simulink model "object_tracker_for_demo"  (Simulink 6.4)
settings: Solver=FixedStepDiscrete  StartTime=0.0  StopTime=inf  RelTol=1e-3
StartFcn:
  | ppo_start
StopFcn:
  | ppo_stop
model workspace: external: M-Code (data not in the file)
undefined symbols (not defined in the file or in its folder): Kanade, line_row, Lucas, Rec, SDTV
libraries: dspmtrx3 x11, viptextngfix x9, vipsnks x5, vipconversions x3, vipanalysis x3, vipgeotforms x3, simulink x2, dspwin32 x1, vipstatistics x1, vipmisc x1, dspindex x1, imaqlib x1
settings Model: Creator=don  LastModifiedBy=Raza  ExtModeAutoUpdateStatusClock=off
settings DataIOCC: LimitDataPoints=off  SaveOutput=off  SignalLogging=off  SaveTime=off  SignalLoggingName=sigsOut
settings OptimizationCC: BufferReusableBoundary=off
settings DebuggingCC: AlgebraicLoopMsg=none  CheckExecutionContextPreStartOutputMsg=on  CheckExecutionContextRuntimeOutputMsg=on  SolverPrmCheckMsg=none  SigSpecEnsureSampleTimeMsg=none  ParameterPrecisionLossMsg=none  BusObjectLabelMismatch=none  StrictBusMsg=None
settings HardwareCC: TargetHWDeviceType=32-bit Generic  ProdEqTarget=off

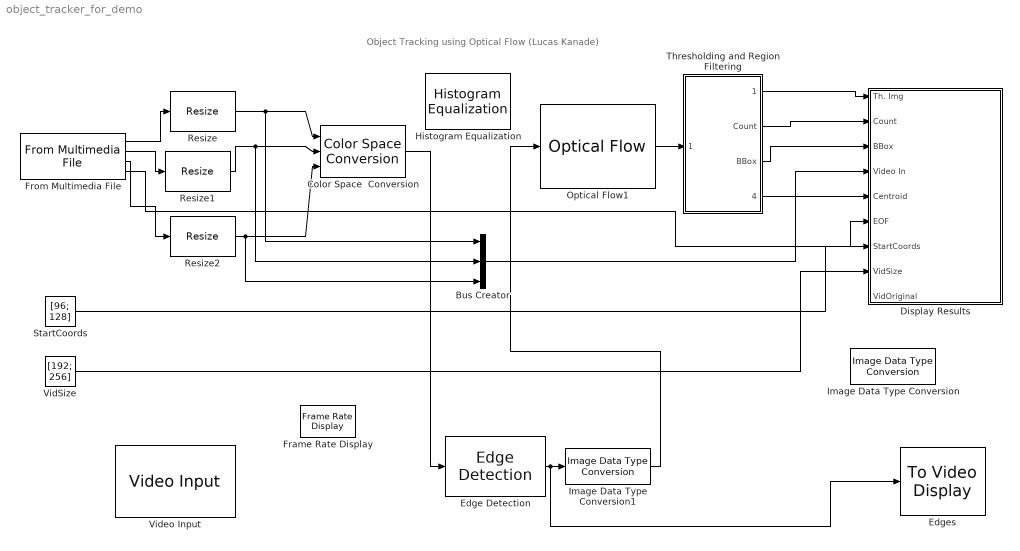
== system object_tracker_for_demo ==
  note: Object Tracking using Optical Flow (Lucas Kanade)
  Bus Creator : BusCreator  Inputs=3
  Color Space  Conversion : vipconversions/Color Space  Conversion  conversion=R'G'B' to intensity  wp_str=D65  rec=Rec. 601 (SDTV)  sys=1125/60/2:1
  Display Results : Subsystem
  Edge Detection : vipanalysis/Edge Detection  DialogController=vipDDGCreate  DialogControllerArgs=DataTag2  method=Prewitt  outputType=Binary image  userDefinedThreshold=on  thresholdSource=Specify via dialog  threshold=0.12  thresholdTuning=10  edgeThinning=off  threshold_canny=[0.25 0.60]  autoPercent=70  sigma=3  roundingMode=Floor  overflowMode=off
  Edges : vipsnks/To Video Display  inputType=Intensity  OutputDevice=On-screen video monitor  fullScreen=off  videoWindowX=692  videoWindowY=89  saveWindowSize=off  videoWindowWidth=264  videoWindowHeight=219
  Frame Rate Display : vipsnks/Frame Rate Display  DialogController=vipDDGCreate  DialogControllerArgs=DataTag3  UpdateRate=10
  From Multimedia File : dspwin32/From Multimedia File  DialogController=dspDDGCreate  DialogControllerArgs=DataTag4  inputFilename=D:\FYP\videos\test-video.mpg  loop=on  numPlays=inf  outputStreams=Video only  videoDataType=single  audioDataType=int16  inheritSampleTime=on  userDefinedSampleTime=1/30  noAudioOutput=off  isIntensityVideo=off  outputEOF=on
  Histogram Equalization : vipanalysis/Histogram Equalization  specify=Uniform  numbins=256  src=Specify via dialog  hist=ones(1,64)
  Image Data Type Conversion : vipconversions/Image Data Type Conversion  outDT=double  isSigned=on  wordLen=16  numFracBits=0
  Image Data Type Conversion1 : vipconversions/Image Data Type Conversion  outDT=single  isSigned=on  wordLen=16  numFracBits=0
  Optical Flow1 : vipanalysis/Optical Flow  SystemSampleTime=-1  method=Lucas-Kanade  which2img=Current frame and N-th frame back  N=1  outVelForm=Magnitude-squared  lambda=1  stop_criteria=When maximum number of iterations is reached  maxAllowAbsDiff=eps  maxIter=10  eigTh=0.01
  Resize : vipgeotforms/Resize  DialogController=vipDDGCreate  DialogControllerArgs=DataTag5  specify=Number of output rows and columns  rfactor=[200 150]  outCols=200  outRows=300  outRowsCols=[192 256]  interp_method=Bilinear  antialias=on  prodOutputMode=Binary point scaling  prodOutputWordLength=32  prodOutputFracLength=10  roundingMode=Nearest  overflowMode=on
  Resize1 : vipgeotforms/Resize  DialogController=vipDDGCreate  DialogControllerArgs=DataTag6  specify=Number of output rows and columns  rfactor=[200 150]  outCols=[300 250]  outRows=300  outRowsCols=[192 256]  interp_method=Nearest neighbor  antialias=on  prodOutputMode=Binary point scaling  prodOutputWordLength=32  prodOutputFracLength=10  roundingMode=Nearest  overflowMode=on
  Resize2 : vipgeotforms/Resize  DialogController=vipDDGCreate  DialogControllerArgs=DataTag7  specify=Number of output rows and columns  rfactor=[200 150]  outCols=200  outRows=300  outRowsCols=[192 256]  interp_method=Nearest neighbor  antialias=on  prodOutputMode=Binary point scaling  prodOutputWordLength=32  prodOutputFracLength=10  roundingMode=Nearest  overflowMode=on
  StartCoords : Constant  Value=[96; 128]  OutDataTypeMode=double  OutDataType=sfix(16)  ConRadixGroup=Use specified scaling  OutScaling=2^0  SampleTime=inf  FramePeriod=inf
      settings: SamplingMode=Frame based
  Thresholding and Region Filtering : Subsystem
  VidSize : Constant  Value=[192; 256]  OutDataTypeMode=double  OutDataType=sfix(16)  ConRadixGroup=Use specified scaling  OutScaling=2^0  SampleTime=inf  FramePeriod=inf
      settings: SamplingMode=Frame based
  Video Input : imaqlib/Video Input  DialogController=imaqcreatedialog  DialogControllerArgs=DataTag9  VideoDeviceMenu=1 (Bt878 TV Card)  VideoDevice=1 (Bt878 TV Card)  VideoStreamFormatMenu=RGB24_768x576  VideoStreamFormat=RGB24_768x576  VideoFrameSizeMenu=INPUTSIZE  VideoFrameSize=INPUTSIZE  FrameRate=30 fps  DataType=double
  wires:
  Thresholding and Region Filtering/3(BBox) -> Display Results/3(BBox)
  Thresholding and Region Filtering/2(Count) -> Display Results/2(Count)
  Bus Creator/1 -> Display Results/4(Video In)
  Thresholding and Region Filtering/4(Centroid) -> Display Results/5(Centroid)
  StartCoords/1 -> Display Results/7(StartCoords)
  VidSize/1 -> Display Results/8(VidSize)
  Optical Flow1/1 -> Thresholding and Region Filtering/1(Sq. Mag)
  Thresholding and Region Filtering/1(Th. Img) -> Display Results/1(Th. Img)
  Edge Detection/1 -> Image Data Type Conversion1/1, Edges/1
  Image Data Type Conversion1/1 -> Optical Flow1/1
  Color Space  Conversion/1 -> Edge Detection/1
  From Multimedia File/1 -> Resize/1
  From Multimedia File/2 -> Resize1/1
  From Multimedia File/3 -> Resize2/1
  Resize/1 -> Color Space  Conversion/1, Bus Creator/1
  Resize1/1 -> Color Space  Conversion/2, Bus Creator/2
  Resize2/1 -> Color Space  Conversion/3, Bus Creator/3
  From Multimedia File/4 -> Display Results/6(EOF)

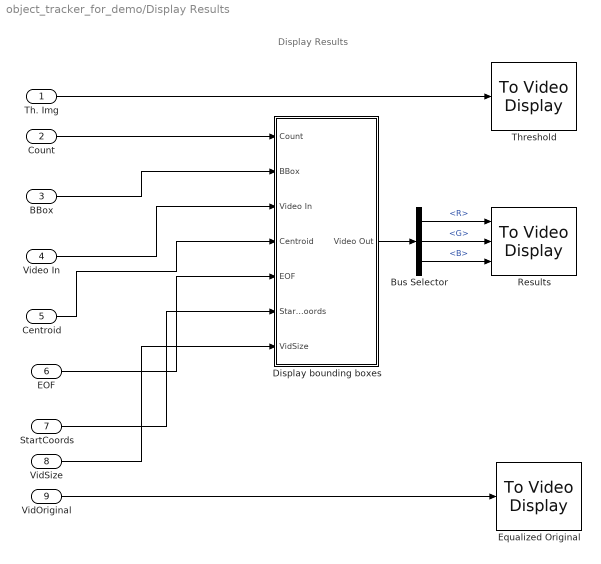
== system object_tracker_for_demo/Display Results ==
  note: Display Results
  Th. Img : Inport
  Count : Inport  Port=2
  BBox : Inport  Port=3
  Video In : Inport  Port=4
  Centroid : Inport  Port=5
  EOF : Inport  Port=6
  StartCoords : Inport  Port=7
  VidSize : Inport  Port=8
  VidOriginal : Inport  Port=9
  Bus Selector : BusSelector  OutputSignals=R,G,B
  Display bounding boxes : Subsystem
  Equalized Original : vipsnks/To Video Display  inputType=Intensity  OutputDevice=On-screen video monitor  fullScreen=off  videoWindowX=172  videoWindowY=305  saveWindowSize=off  videoWindowWidth=112  videoWindowHeight=28
  Results : vipsnks/To Video Display  inputType=RGB  OutputDevice=On-screen video monitor  fullScreen=off  videoWindowX=172  videoWindowY=89  saveWindowSize=off  videoWindowWidth=264  videoWindowHeight=219
  Threshold : vipsnks/To Video Display  inputType=Intensity  OutputDevice=On-screen video monitor  fullScreen=off  videoWindowX=432  videoWindowY=89  saveWindowSize=off  videoWindowWidth=264  videoWindowHeight=219
  wires:
  Bus Selector/1 -> Results/1  "<R>"
  Bus Selector/2 -> Results/2  "<G>"
  Bus Selector/3 -> Results/3  "<B>"
  Th. Img/1 -> Threshold/1
  Count/1 -> Display bounding boxes/1(Count)
  BBox/1 -> Display bounding boxes/2(BBox)
  Centroid/1 -> Display bounding boxes/4(Centroid)
  Display bounding boxes/1(Video Out) -> Bus Selector/1
  Video In/1 -> Display bounding boxes/3(Video In)
  EOF/1 -> Display bounding boxes/5(EOF)
  StartCoords/1 -> Display bounding boxes/6(StartCoords)
  VidSize/1 -> Display bounding boxes/7(VidSize)
  VidOriginal/1 -> Equalized Original/1

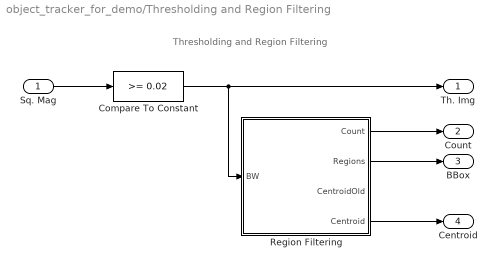
== system object_tracker_for_demo/Thresholding and Region Filtering ==
  note: Thresholding and Region Filtering
  Sq. Mag : Inport
  Compare To Constant : simulink/Logic and Bit Operations/Compare To Constant  SystemSampleTime=-1  relop=>=  const=0.02  LogicOutDataTypeMode=boolean
  Region Filtering : Subsystem
  Th. Img : Outport
  Count : Outport  Port=2
  BBox : Outport  Port=3
  Centroid : Outport  Port=4
  wires:
  Compare To Constant/1 -> Region Filtering/1(BW), Th. Img/1
  Sq. Mag/1 -> Compare To Constant/1
  Region Filtering/1(Count) -> Count/1
  Region Filtering/2(Regions) -> BBox/1
  Region Filtering/4(Centroid) -> Centroid/1

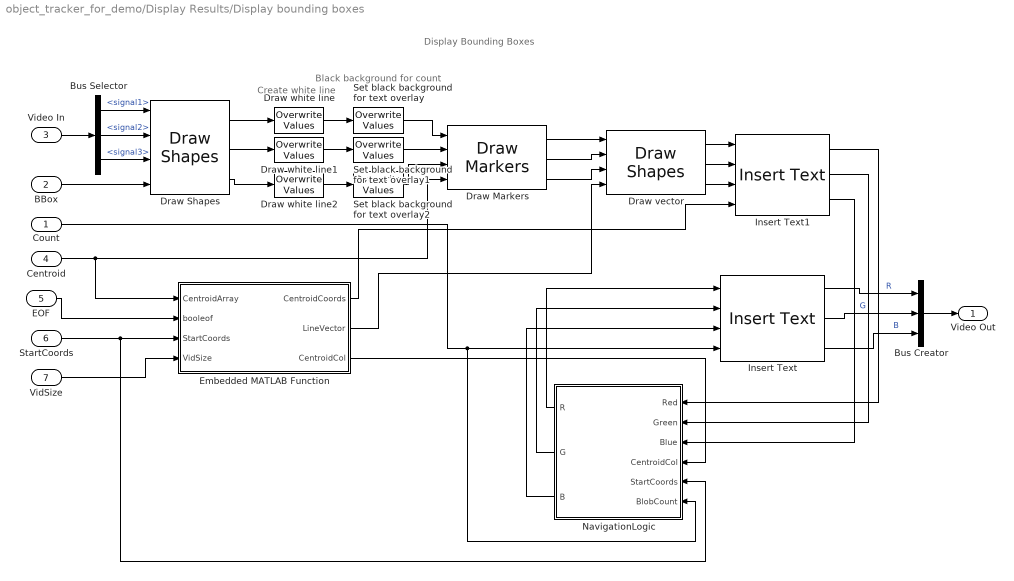
== system object_tracker_for_demo/Display Results/Display bounding boxes ==
  note: Black background
      | for count
  note: Create white
      | line
  note: Display Bounding Boxes
  Count : Inport
  BBox : Inport  Port=2
  Video In : Inport  Port=3
  Centroid : Inport  Port=4
  EOF : Inport  Port=5
  StartCoords : Inport  Port=6
  VidSize : Inport  Port=7
  Bus Creator : BusCreator  Inputs=3
  Bus Selector : BusSelector  OutputSignals=signal1,signal2,signal3
  Draw Markers : viptextngfix/Draw Markers  inType=RGB  shape=X-mark  size=3  fill=off  display=White  intensity=155  color=[200 120 50]  opacity=1  viewport=Entire image
  Draw Shapes : viptextngfix/Draw Shapes  DialogController=vipDDGCreate  DialogControllerArgs=DataTag0  inType=RGB  shape=Rectangles  fill=off  display=User-specified value  intensity=200  color=[0 1 0]  opacity=0.6  viewport=Entire image  antialiasing=off
  Draw vector : viptextngfix/Draw Shapes  DialogController=vipDDGCreate  DialogControllerArgs=DataTag1  inType=RGB  shape=Lines  fill=off  display=White  intensity=200  color=[200 255 100]  opacity=0.6  viewport=Entire image  antialiasing=off
  Draw white line : dspmtrx3/Overwrite Values  OverWriteDiag=Submatrix  valFrom2ndIP=Specify via dialog  ConstValue=1  RowSpan=Range of rows  RowStartMode=Index  RowStartIndex=22  RowEndMode=Index  RowEndIndex=22+1  ColSpan=All columns  ColStartMode=First  ColStartIndex=1  ColEndMode=Last  ColEndIndex=1  DiagSpan=Range of elements  DiagStartMode=Index  DiagStartIndex=2  DiagEndMode=Index  DiagEndIndex=4
  Draw white line1 : dspmtrx3/Overwrite Values  OverWriteDiag=Submatrix  valFrom2ndIP=Specify via dialog  ConstValue=1  RowSpan=Range of rows  RowStartMode=Index  RowStartIndex=22  RowEndMode=Index  RowEndIndex=22+1  ColSpan=All columns  ColStartMode=First  ColStartIndex=1  ColEndMode=Last  ColEndIndex=1  DiagSpan=Range of elements  DiagStartMode=Index  DiagStartIndex=2  DiagEndMode=Index  DiagEndIndex=4
  Draw white line2 : dspmtrx3/Overwrite Values  OverWriteDiag=Submatrix  valFrom2ndIP=Specify via dialog  ConstValue=1  RowSpan=Range of rows  RowStartMode=Index  RowStartIndex=22  RowEndMode=Index  RowEndIndex=22+1  ColSpan=All columns  ColStartMode=First  ColStartIndex=1  ColEndMode=Last  ColEndIndex=1  DiagSpan=Range of elements  DiagStartMode=Index  DiagStartIndex=2  DiagEndMode=Index  DiagEndIndex=4
  Embedded MATLAB Function : Stateflow chart
  Insert Text : viptextngfix/Insert Text  inputType=RGB  theText='%4d'  fontFace=Arial  dummyVar1=0  blockFontSize=12  antiAliased=on  getTextLocFrom=Specify via dialog  textLoc=[0 0]  getTextColorFrom=Specify via dialog  textColor=[1 1 1]  getTextIntensityFrom=Specify via dialog  textIntensity=1  getTextOpacityFrom=Specify via dialog  textOpacity=1.0  dummyVar2=0  dummyVar3=0  dummyVar4=0
  Insert Text1 : viptextngfix/Insert Text  inputType=RGB  theText='(%2.0f,%2.0f)'  fontFace=Arial  dummyVar1=0  blockFontSize=12  antiAliased=on  getTextLocFrom=Specify via dialog  textLoc=[0 40]  getTextColorFrom=Specify via dialog  textColor=[1 1 1]  getTextIntensityFrom=Specify via dialog  textIntensity=1  getTextOpacityFrom=Specify via dialog  textOpacity=1.0  dummyVar2=0  dummyVar3=0  dummyVar4=0
  NavigationLogic : Subsystem  Orientation=left
  Set black background for text overlay : dspmtrx3/Overwrite Values  OverWriteDiag=Submatrix  valFrom2ndIP=Specify via dialog  ConstValue=0  RowSpan=Range of rows  RowStartMode=First  RowStartIndex=25  RowEndMode=Index  RowEndIndex=15  ColSpan=Range of columns  ColStartMode=First  ColStartIndex=1  ColEndMode=Index  ColEndIndex=30  DiagSpan=Range of elements  DiagStartMode=Index  DiagStartIndex=2  DiagEndMode=Index  DiagEndIndex=4
  Set black background for text overlay1 : dspmtrx3/Overwrite Values  OverWriteDiag=Submatrix  valFrom2ndIP=Specify via dialog  ConstValue=0  RowSpan=Range of rows  RowStartMode=First  RowStartIndex=25  RowEndMode=Index  RowEndIndex=15  ColSpan=Range of columns  ColStartMode=First  ColStartIndex=1  ColEndMode=Index  ColEndIndex=30  DiagSpan=Range of elements  DiagStartMode=Index  DiagStartIndex=2  DiagEndMode=Index  DiagEndIndex=4
  Set black background for text overlay2 : dspmtrx3/Overwrite Values  OverWriteDiag=Submatrix  valFrom2ndIP=Specify via dialog  ConstValue=0  RowSpan=Range of rows  RowStartMode=First  RowStartIndex=25  RowEndMode=Index  RowEndIndex=15  ColSpan=Range of columns  ColStartMode=First  ColStartIndex=1  ColEndMode=Index  ColEndIndex=30  DiagSpan=Range of elements  DiagStartMode=Index  DiagStartIndex=2  DiagEndMode=Index  DiagEndIndex=4
  Video Out : Outport
  wires:
  Bus Creator/1 -> Video Out/1
  Draw Shapes/3 -> Draw white line2/1
  Draw Shapes/2 -> Draw white line1/1
  Draw white line2/1 -> Set black background for text overlay2/1
  Draw white line1/1 -> Set black background for text overlay1/1
  Bus Selector/3 -> Draw Shapes/3  "<signal3>"
  Bus Selector/2 -> Draw Shapes/2  "<signal2>"
  Bus Selector/1 -> Draw Shapes/1  "<signal1>"
  Video In/1 -> Bus Selector/1
  BBox/1 -> Draw Shapes/4
  Draw Shapes/1 -> Draw white line/1
  Draw white line/1 -> Set black background for text overlay/1
  Centroid/1 -> Draw Markers/4, Embedded MATLAB Function/1(CentroidArray)
  Set black background for text overlay/1 -> Draw Markers/1
  Set black background for text overlay1/1 -> Draw Markers/2
  Set black background for text overlay2/1 -> Draw Markers/3
  Draw Markers/1 -> Draw vector/1
  Draw Markers/2 -> Draw vector/2
  Draw Markers/3 -> Draw vector/3
  Draw vector/1 -> Insert Text1/1
  Draw vector/2 -> Insert Text1/2
  Draw vector/3 -> Insert Text1/3
  Insert Text1/1 -> NavigationLogic/1(Red)
  Insert Text1/2 -> NavigationLogic/2(Green)
  Insert Text1/3 -> NavigationLogic/3(Blue)
  Embedded MATLAB Function/2(LineVector) -> Draw vector/4
  EOF/1 -> Embedded MATLAB Function/2(booleof)
  StartCoords/1 -> Embedded MATLAB Function/3(StartCoords), NavigationLogic/5(StartCoords)
  VidSize/1 -> Embedded MATLAB Function/4(VidSize)
  Embedded MATLAB Function/3(CentroidCol) -> NavigationLogic/4(CentroidCol)
  Embedded MATLAB Function/1(CentroidCoords) -> Insert Text1/4
  Insert Text/1 -> Bus Creator/1  "R"
  Insert Text/2 -> Bus Creator/2  "G"
  Insert Text/3 -> Bus Creator/3  "B"
  Count/1 -> Insert Text/4, NavigationLogic/6(BlobCount)
  NavigationLogic/1(R) -> Insert Text/1
  NavigationLogic/2(G) -> Insert Text/2
  NavigationLogic/3(B) -> Insert Text/3

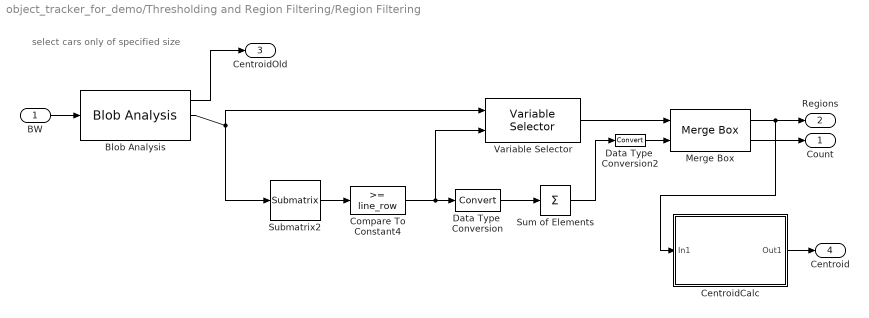
== system object_tracker_for_demo/Thresholding and Region Filtering/Region Filtering ==
  note: select cars only of specified size
  BW : Inport
  Blob Analysis : vipstatistics/Blob Analysis  DialogController=vipDDGCreate  DialogControllerArgs=DataTag8  area=off  centroid=on  bBox=on  majorAxis=off  minorAxis=off  angle=off  eccentricity=off  equivDiameterSq=off  extent=off  perimeter=off  maxBlobs=10  warnIfNumBlobsExceeded=on  isCount=on  useMinArea=on  minArea=100  useMaxArea=on  maxArea=2500  excludeBorderBlob=off  outDT=single  isFill=on  fillValues=-1  conn=8  isLabel=off  outputMode=Binary point scaling  outputWordLength=32  outputFracLength=16  firstCoeffMode=Binary point scaling  firstCoeffWordLength=16  firstCoeffFracLength=14  secondCoeffMode=Binary point scaling  secondCoeffWordLength=32  secondCoeffFracLength=16  accumMode=Binary point scaling  accumWordLength=32  accumFracLength=0  prodOutputMode=Binary point scaling  prodOutputWordLength=32  prodOutputFracLength=16  roundingMode=Floor  overflowMode=off
  CentroidCalc : Subsystem
  Compare To Constant4 : simulink/Logic and Bit Operations/Compare To Constant  SystemSampleTime=-1  relop=>=  const=line_row  LogicOutDataTypeMode=boolean  ZeroCross=off
  Data Type  Conversion : DataTypeConversion  OutDataTypeMode=single  SaturateOnIntegerOverflow=on  RndMeth=Zero
  Data Type  Conversion2 : DataTypeConversion  OutDataTypeMode=int32  SaturateOnIntegerOverflow=on  RndMeth=Zero
  Merge Box : vipmisc/Merge Box  whichdir=Row direction only  cdist=60  rdist=45
  Submatrix2 : dspmtrx3/Submatrix  RowSpan=One row  RowStartMode=Index  RowStartIndex=1  RowEndMode=Last  RowEndIndex=1  ColSpan=All columns  ColStartMode=First  ColStartIndex=1  ColEndMode=Last  ColEndIndex=1
  Sum of Elements : Sum  Inputs=+  OutScaling=2^-10
  Variable Selector : dspindex/Variable Selector  NumInputs=1  rowsOrCols=Columns  IdxMode=Variable  Elements=[1 3]  ZerOneIdxMode=Zero-based  errmode=Clip Index  FillMode=on  FillValues=-1
  Count : Outport
  Regions : Outport  Port=2
  CentroidOld : Outport  Port=3
  Centroid : Outport  Port=4
  wires:
  Data Type  Conversion/1 -> Sum of Elements/1
  Sum of Elements/1 -> Data Type  Conversion2/1
  Compare To Constant4/1 -> Data Type  Conversion/1, Variable Selector/2
  Submatrix2/1 -> Compare To Constant4/1
  BW/1 -> Blob Analysis/1
  Variable Selector/1 -> Merge Box/1
  Merge Box/1 -> Regions/1, CentroidCalc/1(In1)
  Merge Box/2 -> Count/1
  Data Type  Conversion2/1 -> Merge Box/2
  Blob Analysis/2 -> Submatrix2/1, Variable Selector/1
  Blob Analysis/1 -> CentroidOld/1
  CentroidCalc/1(Out1) -> Centroid/1

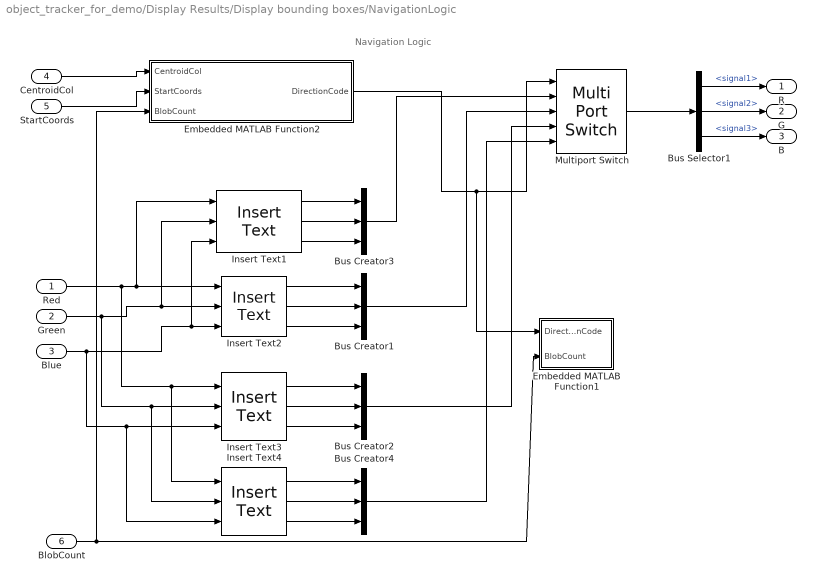
== system object_tracker_for_demo/Display Results/Display bounding boxes/NavigationLogic ==
  note: Navigation Logic
  Red : Inport
  Green : Inport  Port=2
  Blue : Inport  Port=3
  CentroidCol : Inport  Port=4
  StartCoords : Inport  Port=5
  BlobCount : Inport  Port=6
  Bus Creator{1..4} (4 alike) : BusCreator  Inputs=3
  Bus Selector1 : BusSelector  OutputSignals=signal1,signal2,signal3
  Embedded MATLAB Function1 : Stateflow chart
  Embedded MATLAB Function2 : Stateflow chart
  Insert Text1 : viptextngfix/Insert Text  inputType=RGB  theText='STRAIGHT'  fontFace=Arial  dummyVar1=0  blockFontSize=12  antiAliased=on  getTextLocFrom=Specify via dialog  textLoc=[0 100]  getTextColorFrom=Specify via dialog  textColor=[1 1 1]  getTextIntensityFrom=Specify via dialog  textIntensity=1  getTextOpacityFrom=Specify via dialog  textOpacity=1.0  dummyVar2=0  dummyVar3=0  dummyVar4=0
  Insert Text2 : viptextngfix/Insert Text  inputType=RGB  theText='LEFT'  fontFace=Arial  dummyVar1=0  blockFontSize=12  antiAliased=on  getTextLocFrom=Specify via dialog  textLoc=[0 100]  getTextColorFrom=Specify via dialog  textColor=[1 1 1]  getTextIntensityFrom=Specify via dialog  textIntensity=1  getTextOpacityFrom=Specify via dialog  textOpacity=1.0  dummyVar2=0  dummyVar3=0  dummyVar4=0
  Insert Text3 : viptextngfix/Insert Text  inputType=RGB  theText='RIGHT'  fontFace=Arial  dummyVar1=0  blockFontSize=12  antiAliased=on  getTextLocFrom=Specify via dialog  textLoc=[0 100]  getTextColorFrom=Specify via dialog  textColor=[1 1 1]  getTextIntensityFrom=Specify via dialog  textIntensity=1  getTextOpacityFrom=Specify via dialog  textOpacity=1.0  dummyVar2=0  dummyVar3=0  dummyVar4=0
  Insert Text4 : viptextngfix/Insert Text  inputType=RGB  theText='STOP'  fontFace=Arial  dummyVar1=0  blockFontSize=12  antiAliased=on  getTextLocFrom=Specify via dialog  textLoc=[0 100]  getTextColorFrom=Specify via dialog  textColor=[1 1 1]  getTextIntensityFrom=Specify via dialog  textIntensity=1  getTextOpacityFrom=Specify via dialog  textOpacity=1.0  dummyVar2=0  dummyVar3=0  dummyVar4=0
  Multiport Switch : MultiPortSwitch
  R : Outport
  G : Outport  Port=2
  B : Outport  Port=3
  wires:
  Bus Selector1/1 -> R/1  "<signal1>"
  Bus Selector1/2 -> G/1  "<signal2>"
  Bus Selector1/3 -> B/1  "<signal3>"
  Bus Creator1/1 -> Multiport Switch/3
  Bus Creator2/1 -> Multiport Switch/4
  Red/1 -> Insert Text2/1, Insert Text1/1, Insert Text3/1, Insert Text4/1
  Green/1 -> Insert Text2/2, Insert Text1/2, Insert Text3/2, Insert Text4/2
  Blue/1 -> Insert Text2/3, Insert Text1/3, Insert Text3/3, Insert Text4/3
  Insert Text2/1 -> Bus Creator1/1
  Insert Text2/2 -> Bus Creator1/2
  Insert Text2/3 -> Bus Creator1/3
  Insert Text3/1 -> Bus Creator2/1
  Insert Text3/2 -> Bus Creator2/2
  Insert Text3/3 -> Bus Creator2/3
  Multiport Switch/1 -> Bus Selector1/1
  Insert Text1/1 -> Bus Creator3/1
  Insert Text1/2 -> Bus Creator3/2
  Insert Text1/3 -> Bus Creator3/3
  Bus Creator3/1 -> Multiport Switch/2
  CentroidCol/1 -> Embedded MATLAB Function2/1(CentroidCol)
  StartCoords/1 -> Embedded MATLAB Function2/2(StartCoords)
  Embedded MATLAB Function2/1(DirectionCode) -> Multiport Switch/1, Embedded MATLAB Function1/1(DirectionCode)
  BlobCount/1 -> Embedded MATLAB Function1/2(BlobCount), Embedded MATLAB Function2/3(BlobCount)
  Insert Text4/1 -> Bus Creator4/1
  Insert Text4/2 -> Bus Creator4/2
  Insert Text4/3 -> Bus Creator4/3
  Bus Creator4/1 -> Multiport Switch/5

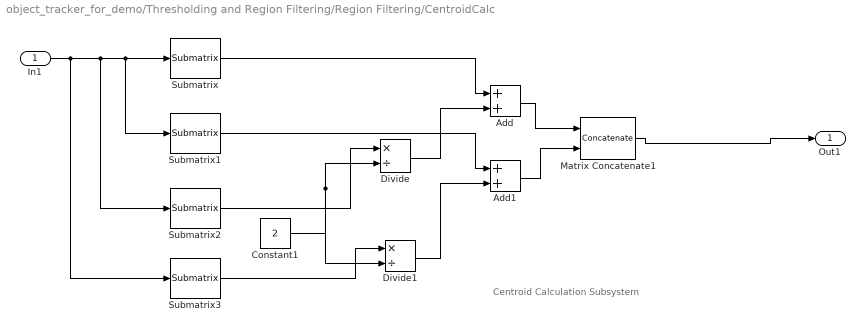
== system object_tracker_for_demo/Thresholding and Region Filtering/Region Filtering/CentroidCalc ==
  note: Centroid Calculation
      | Subsystem
  In1 : Inport
  Add : Sum  OutScaling=2^-10
  Add1 : Sum  OutScaling=2^-10
  Constant1 : Constant  Value=2  OutDataType=sfix(16)  ConRadixGroup=Use specified scaling  OutScaling=2^0  SampleTime=inf  FramePeriod=inf
  Divide : Product  Inputs=*/  OutScaling=2^-10
  Divide1 : Product  Inputs=*/  OutScaling=2^-10
  Matrix Concatenate1 : Concatenate  Mode=Vertical matrix concatenation
  Submatrix : dspmtrx3/Submatrix  RowSpan=One row  RowStartMode=Index  RowStartIndex=1  RowEndMode=Last  RowEndIndex=1  ColSpan=All columns  ColStartMode=Offset from last  ColStartIndex=1  ColEndMode=Last  ColEndIndex=1
  Submatrix1 : dspmtrx3/Submatrix  RowSpan=One row  RowStartMode=Index  RowStartIndex=2  RowEndMode=Last  RowEndIndex=1  ColSpan=All columns  ColStartMode=Offset from last  ColStartIndex=1  ColEndMode=Last  ColEndIndex=1
  Submatrix2 : dspmtrx3/Submatrix  RowSpan=One row  RowStartMode=Index  RowStartIndex=3  RowEndMode=Last  RowEndIndex=1  ColSpan=All columns  ColStartMode=Offset from last  ColStartIndex=1  ColEndMode=Last  ColEndIndex=1
  Submatrix3 : dspmtrx3/Submatrix  RowSpan=One row  RowStartMode=Index  RowStartIndex=4  RowEndMode=Last  RowEndIndex=1  ColSpan=All columns  ColStartMode=Offset from last  ColStartIndex=1  ColEndMode=Last  ColEndIndex=1
  Out1 : Outport
  wires:
  Add1/1 -> Matrix Concatenate1/2
  Add/1 -> Matrix Concatenate1/1
  Divide1/1 -> Add1/2
  Submatrix1/1 -> Add1/1
  Divide/1 -> Add/2
  Submatrix/1 -> Add/1
  Submatrix3/1 -> Divide1/1
  Submatrix2/1 -> Divide/1
  Constant1/1 -> Divide/2, Divide1/2
  In1/1 -> Submatrix/1, Submatrix1/1, Submatrix2/1, Submatrix3/1
  Matrix Concatenate1/1 -> Out1/1

== matlab function Display Results/Display bounding boxes/NavigationLogic/Embedded MATLAB Function1 ==
  data: DirectionCode input inherited; BlobCount input inherited
function Turnit(DirectionCode, BlobCount)
% This block supports an embeddable subset of the MATLAB language.
% See the help menu for details. 
DIFFTHING = 5;
BRAKEDIFF = 2;

persistent movecount; %no of frames after which the position of the car is updated.
persistent brakecount;

persistent startflag;

if isempty ( startflag ) 
    startflag = 1;
else
    startflag = 0;
end

if isempty ( brakecount ) 
    brakecount = 0;
end

if  isempty ( movecount ) 
    movecount = 0;
end

if BlobCount == 0 
    movecount = DIFFTHING;
    brakecount = 0;
    startflag = 1;
    BrakeAll;
    return;
end

movecount = movecount + 1;
brakecount = brakecount + 1;

if ( brakecount >= BRAKEDIFF )
    BrakeAll;
end

    
if ( movecount >= DIFFTHING || startflag == 1 )
    
    if  DirectionCode == 1    %Forward
        MoveForward(1);
    elseif  DirectionCode == 2  %Left
        MoveLeft ( 1 );
    elseif DirectionCode == 3  %Right
        MoveRight ( 1 );
    end

    MoveForward(1);
    movecount = 0;

end

== matlab function Display Results/Display bounding boxes/Embedded MATLAB Function ==
  data: CentroidCoords output inherited; CentroidArray input inherited; LineVector output inherited; booleof input inherited; StartCoords input inherited; VidSize input inherited; CentroidCol output inherited
function [CentroidCoords,LineVector, CentroidCol] = ObjectTracker(CentroidArray,booleof,StartCoords,VidSize)
% This block supports an embeddable subset of the MATLAB language.
% See the help menu for details. 
persistent LastCentroid;

if isempty(LastCentroid) || booleof == true
    LastCentroid = StartCoords;
end

z = LastCentroid;

allx = CentroidArray(1,:) - z(1);
ally = CentroidArray(2,:) - z(2);
myvector =  sqrt(allx.^2 + ally.^2);
[m i] = min (myvector);
centroid = CentroidArray(:,i(1));

if myvector(i(1)) < 100 && centroid(1) > 0 && centroid(2) > 10
    LastCentroid = centroid;
    CentroidCoords = centroid;
else
    CentroidCoords = z;
end

LineVector = [ VidSize(1) , VidSize(2)/2 , CentroidCoords(1) , CentroidCoords(2) ];
CentroidCol = CentroidCoords(2);

== matlab function Display Results/Display bounding boxes/NavigationLogic/Embedded MATLAB Function2 ==
  data: CentroidCol input inherited; StartCoords input inherited; DirectionCode output inherited; BlobCount input inherited
function DirectionCode = DirectionTest(CentroidCol, StartCoords, BlobCount)

STRAIGHT = 1;
LEFT = 2;
RIGHT = 3;
STOP = 4;

DIFFTHRESHOLD = 20;
ScreenCenter = StartCoords(2);

if BlobCount == 0
    DirectionCode = STOP;
elseif CentroidCol < ScreenCenter - DIFFTHRESHOLD
    DirectionCode = LEFT;
elseif CentroidCol > ScreenCenter + DIFFTHRESHOLD
    DirectionCode = RIGHT;
else
    DirectionCode = STRAIGHT;
end
